simulink model "fz8_13"  (R2014a)
settings: Solver=ode45  StartTime=0.0  StopTime=10.0  RelTol=1e-3
undefined symbols (not defined in the file or in its folder): gfprimfd
libraries: commblkcod2 x3, commsink2 x2, commblkintrlv2 x2, commrandsrc2 x1
settings Model: Creator=tzb  LastModifiedBy=tzb

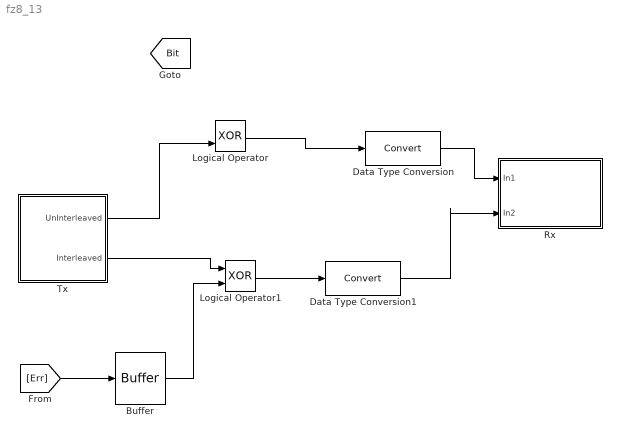
== system fz8_13 ==
  Buffer : Buffer  N=30*20  TreatMby1Signals=One channel
  Data Type Conversion : DataTypeConversion
  Data Type Conversion1 : DataTypeConversion
  Logical Operator : Logic  Operator=XOR  AllPortsSameDT=off  OutDataTypeStr=boolean
  Logical Operator1 : Logic  Operator=XOR  AllPortsSameDT=off  OutDataTypeStr=boolean
  Rx : Subsystem
  Tx : Subsystem
  tag scope: Bit=global
  wires:
  Tx/1(UnInterleaved) -> Logical Operator/2
  Tx/2(Interleaved) -> Logical Operator1/1
  [Err] -> Buffer/1
  Buffer/1 -> Logical Operator1/2
  Logical Operator1/1 -> Data Type Conversion1/1
  Logical Operator/1 -> Data Type Conversion/1
  Data Type Conversion/1 -> Rx/1(In1)
  Data Type Conversion1/1 -> Rx/2(In2)

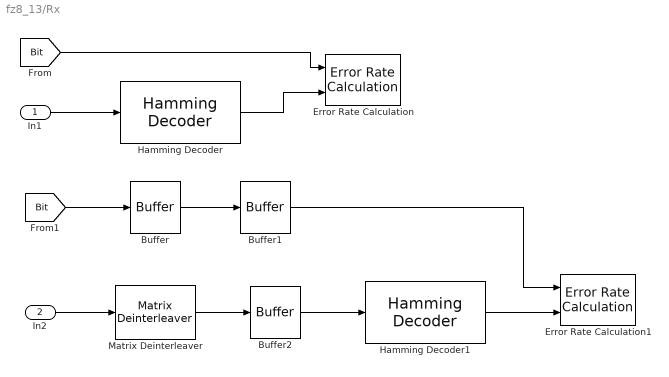
== system fz8_13/Rx ==
  In1 : Inport
  In2 : Inport  Port=2
  Buffer : Buffer  N=440  TreatMby1Signals=One channel
  Buffer1 : Buffer  N=11  TreatMby1Signals=One channel
  Buffer2 : Buffer  N=15  TreatMby1Signals=One channel
  Error Rate Calculation : commsink2/Error Rate Calculation  N=0  st_delay=0  cp_mode=Entire frame  subframe=[]  PMode=Workspace  WsName=BER2  RsMode2=off  stop=off  numErr=100  maxBits=1e6
  Error Rate Calculation1 : commsink2/Error Rate Calculation  N=0  st_delay=440  cp_mode=Entire frame  subframe=[]  PMode=Workspace  WsName=BER1  RsMode2=off  stop=off  numErr=100  maxBits=1e6
  Hamming Decoder : commblkcod2/Hamming Decoder  n=15  k=gfprimfd(4,'min')
  Hamming Decoder1 : commblkcod2/Hamming Decoder  n=15  k=gfprimfd(4,'min')
  Matrix Deinterleaver : commblkintrlv2/Matrix Deinterleaver  Nrows=30  Ncols=20
  wires:
  Buffer2/1 -> Hamming Decoder1/1
  Buffer1/1 -> Error Rate Calculation1/1
  In1/1 -> Hamming Decoder/1
  Hamming Decoder/1 -> Error Rate Calculation/2
  [Bit] -> Error Rate Calculation/1
  In2/1 -> Matrix Deinterleaver/1
  Buffer/1 -> Buffer1/1
  [Bit] -> Buffer/1
  Matrix Deinterleaver/1 -> Buffer2/1
  Hamming Decoder1/1 -> Error Rate Calculation1/2

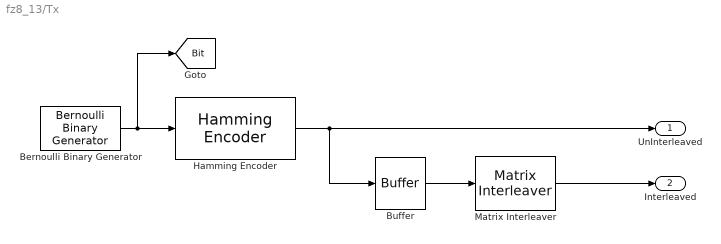
== system fz8_13/Tx ==
  Bernoulli Binary Generator : commrandsrc2/Bernoulli Binary Generator  P=0.5  seed=61  Ts=1/110000  frameBased=on  sampPerFrame=11  orient=off  outDataType=double
  Buffer : Buffer  N=30*20  TreatMby1Signals=One channel
  Hamming Encoder : commblkcod2/Hamming Encoder  n=15  k=gfprimfd(4,'min')
  Matrix Interleaver : commblkintrlv2/Matrix Interleaver  Nrows=30  Ncols=20
  UnInterleaved : Outport
  Interleaved : Outport  Port=2
  tag scope: Bit=global
  wires:
  Bernoulli Binary Generator/1 -> [Bit], Hamming Encoder/1
  Matrix Interleaver/1 -> Interleaved/1
  Hamming Encoder/1 -> UnInterleaved/1, Buffer/1
  Buffer/1 -> Matrix Interleaver/1
